simulink model "Torque_Vectoring_Testing"  (R2024a)
settings: Solver=FixedStepAuto  StartTime=1020  StopTime=1120  FixedStep=0.01  RelTol=1e-3
settings Model: Creator=andre  LastModifiedBy=pedro

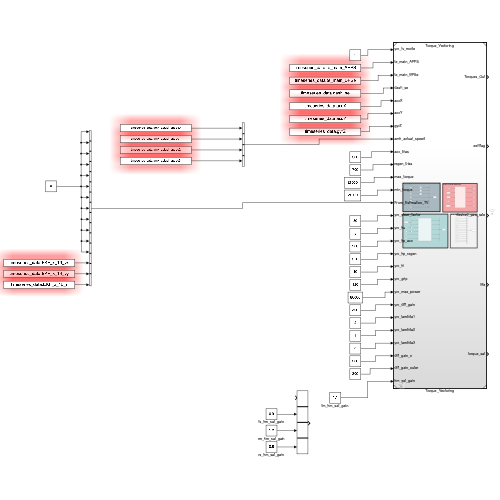
[thumbnail: Simulink's stored preview of the top-level diagram]
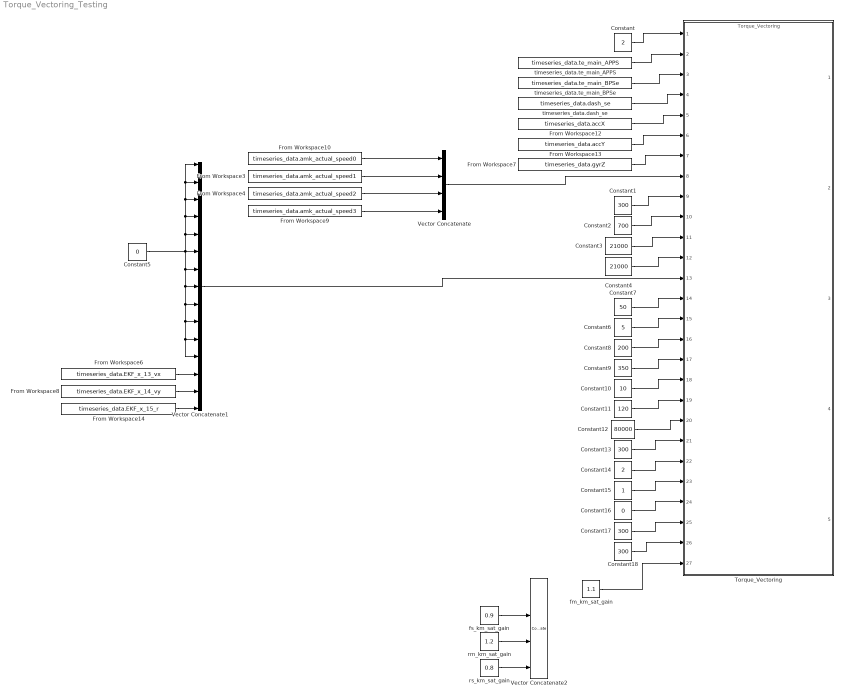
== system Torque_Vectoring_Testing ==
  Constant : Constant  Value=2
  Constant{1,13,17..18} (4 alike) : Constant  Value=300
  Constant10 : Constant  Value=10
  Constant11 : Constant  Value=120
  Constant12 : Constant  Value=80000
  Constant14 : Constant  Value=2
  Constant15 : Constant
  Constant16 : Constant  Value=0
  Constant2 : Constant  Value=700
  Constant3 : Constant  Value=21000
  Constant4 : Constant  Value=21000
  Constant5 : Constant  Value=0
  Constant6 : Constant  Value=5
  Constant7 : Constant  Value=50
  Constant8 : Constant  Value=200
  Constant9 : Constant  Value=350
  From Workspace10 : FromWorkspace  VariableName=timeseries_data.amk_actual_speed0  OutputAfterFinalValue=Setting to zero
  From Workspace12 : FromWorkspace  VariableName=timeseries_data.accX  OutputAfterFinalValue=Setting to zero
  From Workspace13 : FromWorkspace  VariableName=timeseries_data.accY  OutputAfterFinalValue=Setting to zero
  From Workspace14 : FromWorkspace  VariableName=timeseries_data.EKF_x_15_r  OutputAfterFinalValue=Setting to zero
  From Workspace3 : FromWorkspace  VariableName=timeseries_data.amk_actual_speed1  OutputAfterFinalValue=Setting to zero
  From Workspace4 : FromWorkspace  VariableName=timeseries_data.amk_actual_speed2  OutputAfterFinalValue=Setting to zero
  From Workspace6 : FromWorkspace  VariableName=timeseries_data.EKF_x_13_vx  OutputAfterFinalValue=Setting to zero
  From Workspace7 : FromWorkspace  VariableName=timeseries_data.gyrZ  OutputAfterFinalValue=Setting to zero
  From Workspace8 : FromWorkspace  VariableName=timeseries_data.EKF_x_14_vy  OutputAfterFinalValue=Setting to zero
  From Workspace9 : FromWorkspace  VariableName=timeseries_data.amk_actual_speed3  OutputAfterFinalValue=Setting to zero
  Torque_Vectoring : ModelReference  ModelNameDialog=Torque_Vectoring.slx  SimulationMode=Normal  ModelReferenceVersion=4.6
  Vector Concatenate : Concatenate  NumInputs=4
  Vector Concatenate1 : Concatenate  NumInputs=15
  Vector Concatenate2 : Concatenate  NumInputs=4
  fm_km_sat_gain : Constant  Value=1.1
  fs_km_sat_gain : Constant  Value=0.9
  rm_km_sat_gain : Constant  Value=1.2
  rs_km_sat_gain : Constant  Value=0.8
  timeseries_data.dash_se : FromWorkspace  VariableName=timeseries_data.dash_se  OutputAfterFinalValue=Setting to zero
  timeseries_data.te_main_APPS : FromWorkspace  VariableName=timeseries_data.te_main_APPS  OutputAfterFinalValue=Setting to zero
  timeseries_data.te_main_BPSe : FromWorkspace  VariableName=timeseries_data.te_main_BPSe  OutputAfterFinalValue=Setting to zero
  wires:
  Constant10/1 -> Torque_Vectoring/18
  Constant6/1 -> Torque_Vectoring/15
  Constant7/1 -> Torque_Vectoring/14
  timeseries_data.te_main_BPSe/1 -> Torque_Vectoring/3
  From Workspace14/1 -> Vector Concatenate1/15
  From Workspace9/1 -> Vector Concatenate/4
  timeseries_data.te_main_APPS/1 -> Torque_Vectoring/2
  Constant4/1 -> Torque_Vectoring/12
  From Workspace8/1 -> Vector Concatenate1/14
  timeseries_data.dash_se/1 -> Torque_Vectoring/4
  From Workspace12/1 -> Torque_Vectoring/5
  From Workspace7/1 -> Torque_Vectoring/7
  From Workspace13/1 -> Torque_Vectoring/6
  From Workspace10/1 -> Vector Concatenate/1
  From Workspace4/1 -> Vector Concatenate/3
  Constant2/1 -> Torque_Vectoring/10
  Vector Concatenate1/1 -> Torque_Vectoring/13
  Constant13/1 -> Torque_Vectoring/21
  Constant/1 -> Torque_Vectoring/1
  From Workspace3/1 -> Vector Concatenate/2
  Constant1/1 -> Torque_Vectoring/9
  Vector Concatenate/1 -> Torque_Vectoring/8
  Constant3/1 -> Torque_Vectoring/11
  Constant9/1 -> Torque_Vectoring/17
  Constant5/1 -> Vector Concatenate1/1, Vector Concatenate1/2, Vector Concatenate1/3, Vector Concatenate1/4, Vector Concatenate1/5, Vector Concatenate1/12, Vector Concatenate1/11, Vector Concatenate1/10, Vector Concatenate1/9, Vector Concatenate1/8, Vector Concatenate1/7, Vector Concatenate1/6
  Constant12/1 -> Torque_Vectoring/20
  Constant11/1 -> Torque_Vectoring/19
  Constant8/1 -> Torque_Vectoring/16
  From Workspace6/1 -> Vector Concatenate1/13
  Constant14/1 -> Torque_Vectoring/22
  Constant15/1 -> Torque_Vectoring/23
  Constant16/1 -> Torque_Vectoring/24
  Constant18/1 -> Torque_Vectoring/26
  Constant17/1 -> Torque_Vectoring/25
  rs_km_sat_gain/1 -> Vector Concatenate2/4
  fm_km_sat_gain/1 -> Torque_Vectoring/27
  fs_km_sat_gain/1 -> Vector Concatenate2/2
  rm_km_sat_gain/1 -> Vector Concatenate2/3
